simulink model "scheda_analogica_i"  (R2021a)
settings: Solver=VariableStepAuto  StartTime=0.0  StopTime=0.2  RelTol=1e-3
values from neighbouring files (symbols this model uses):
  R = 10e3    (= 10000)    [init_data.m]
  Rburden = 6.6/(1000/3000)    (= 19.8)    [init_data.m]
libraries: fl_lib x132, nesl_utility x23, ee_lib x4
settings Model: Creator=dbagn  LastModifiedBy=dbagn

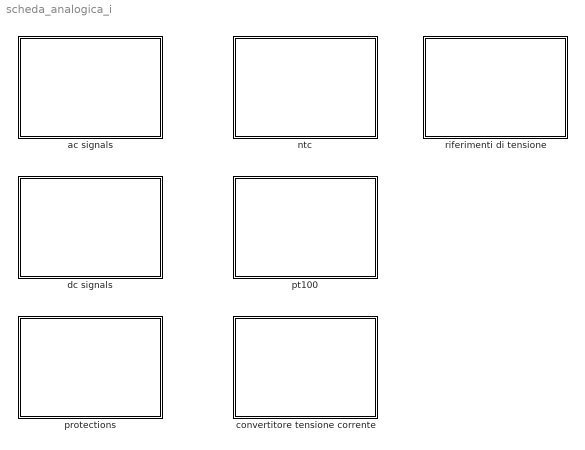
== system scheda_analogica_i ==
  ac signals : Subsystem
  convertitore tensione corrente : Subsystem
  dc signals : Subsystem
  ntc : Subsystem
  protections : Subsystem
  pt100 : Subsystem
  riferimenti di tensione : Subsystem

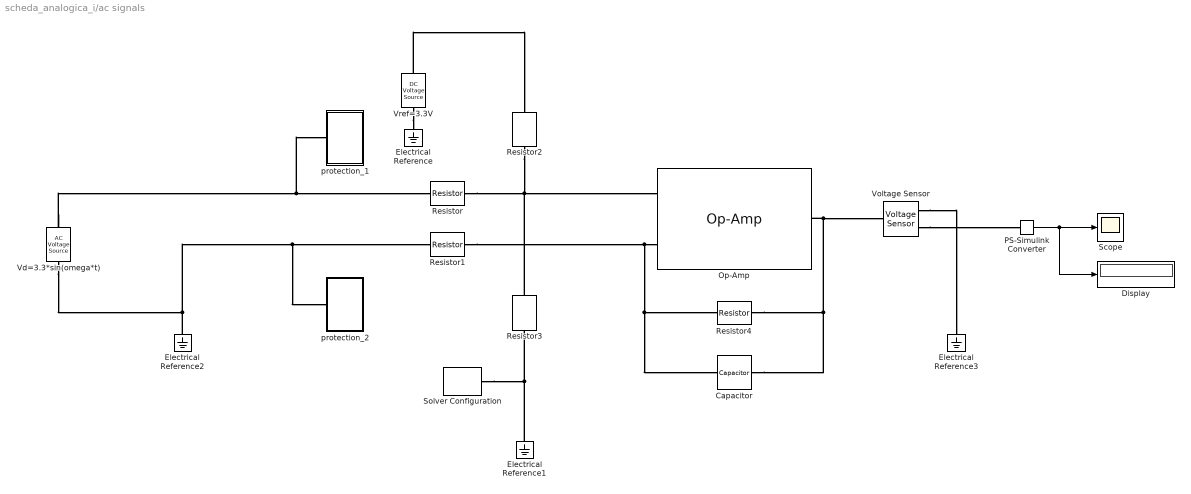
== system scheda_analogica_i/ac signals ==
  Capacitor : fl_lib/Electrical/Electrical Elements/Capacitor  c=47e-12 F  r=0 Ohm  g=0 1/Ohm  i_specify=off  i_priority=None  i=0 A  i_nominal_specify=off  i_nominal_unit=A  i_nominal_value=1  v_specify=off  v_priority=None  v=0 V  v_nominal_specify=off  v_nominal_unit=V  v_nominal_value=1  vc_specify=off  vc_priority=High  vc=0 V  vc_nominal_specify=off  vc_nominal_unit=V  vc_nominal_value=1
  Display : Display
      settings: Decimation=3
  Electrical Reference{,1..3} (4 alike) : fl_lib/Electrical/Electrical Elements/Electrical Reference
  Op-Amp : fl_lib/Electrical/Electrical Elements/Op-Amp  outI_specify=off  outI_priority=None  outI=0 A  outI_nominal_specify=off  outI_nominal_unit=A  outI_nominal_value=1
  PS-Simulink Converter : nesl_utility/PS-Simulink Converter  PhysicalDomain=network_engine_domain  SubClassName=ps_output  LeftPortType=input  RightPortType=output  PseudoPeriodic=off  Frequencies=[]  Unit=V  AffineConversion=on
      settings: SourceProductBaseCode=PW,SS
  Resistor{,1..3} (4 alike) : fl_lib/Electrical/Electrical Elements/Resistor  R=2*R Ohm  i_specify=off  i_priority=None  i=0 A  i_nominal_specify=off  i_nominal_unit=A  i_nominal_value=1  v_specify=off  v_priority=None  v=0 V  v_nominal_specify=off  v_nominal_unit=V  v_nominal_value=1
  Resistor4 : fl_lib/Electrical/Electrical Elements/Resistor  R=R Ohm  i_specify=off  i_priority=None  i=0 A  i_nominal_specify=off  i_nominal_unit=A  i_nominal_value=1  v_specify=off  v_priority=None  v=0 V  v_nominal_specify=off  v_nominal_unit=V  v_nominal_value=1
  Scope : Scope
  Solver Configuration : nesl_utility/Solver Configuration  PhysicalDomain=network_engine_domain  SubClassName=solver  LeftPortType=input  RightPortType=generic  Tones=[]  Harmonics=[]  SimulateNoise=off  Profile=off  UseLocalSampling=off  EnableSwitchedLinearOptims=on  FrequencyDomain=off  UseCCode=off  RelTol=0.001  AbsTol=1e-06  MinStep=1e-09  ToWorkspace=off  RevertToSquareIcSolve=off  NumHomotopyIterations=100  PhasorMode=off  PhasorModeNumHarmonics=1  DoDC=off  ResidualTolerance=1e-09  UseLocalSolver=off  LocalSolverChoice=NE_BACKWARD_EULER_ADVANCER  LocalSolverSampleTime=0.001  DoFixedCost=off  MaxNonlinIter=3  MaxModeIter=2  ComputeImpulses=off  ImpulseIterations=2  LinearAlgebra=auto  EquationFormulation=NE_TIME_EF  DelaysMemoryBudget=1024  AutomaticFiltering=on  FilteringTimeConstant=0.001  PartitionStorageMethod=AS_NEEDED  PartitionMemoryBudget=1024  PartitionMethod=ROBUST
      settings: SourceProductBaseCode=PW,SS
  Vd=3.3*sin(omega*t) : fl_lib/Electrical/Electrical Sources/AC Voltage Source  amp=3.3 V  shift=0 deg  frequency=50 Hz  omega=0 rad/s
  Voltage Sensor : fl_lib/Electrical/Electrical Sensors/Voltage Sensor
  Vref=3.3V : fl_lib/Electrical/Electrical Sources/DC Voltage Source  v0=3.3 V
  protection_1 : Subsystem
  protection_2 : Subsystem
  wires:
  PS-Simulink Converter/1 -> Display/1, Scope/1
  connections:
  Resistor1/RConn1 -- Capacitor/LConn1 -- Resistor4/LConn1 -- Op-Amp/LConn2
  Electrical Reference1/LConn1 -- Solver Configuration/RConn1 -- Resistor3/RConn1
  Vref=3.3V/LConn1 -- Resistor2/LConn1
  Voltage Sensor/RConn1 -- PS-Simulink Converter/LConn1
  Resistor4/RConn1 -- Op-Amp/RConn1 -- Voltage Sensor/LConn1 -- Capacitor/RConn1
  Voltage Sensor/RConn2 -- Electrical Reference3/LConn1
  Resistor3/LConn1 -- Op-Amp/LConn1 -- Resistor2/RConn1 -- Resistor/RConn1
  Vref=3.3V/RConn1 -- Electrical Reference/LConn1
  Vd=3.3*sin(omega*t)/LConn1 -- protection_1/LConn1 -- Resistor/LConn1
  Electrical Reference2/LConn1 -- Vd=3.3*sin(omega*t)/RConn1 -- protection_2/LConn1 -- Resistor1/LConn1

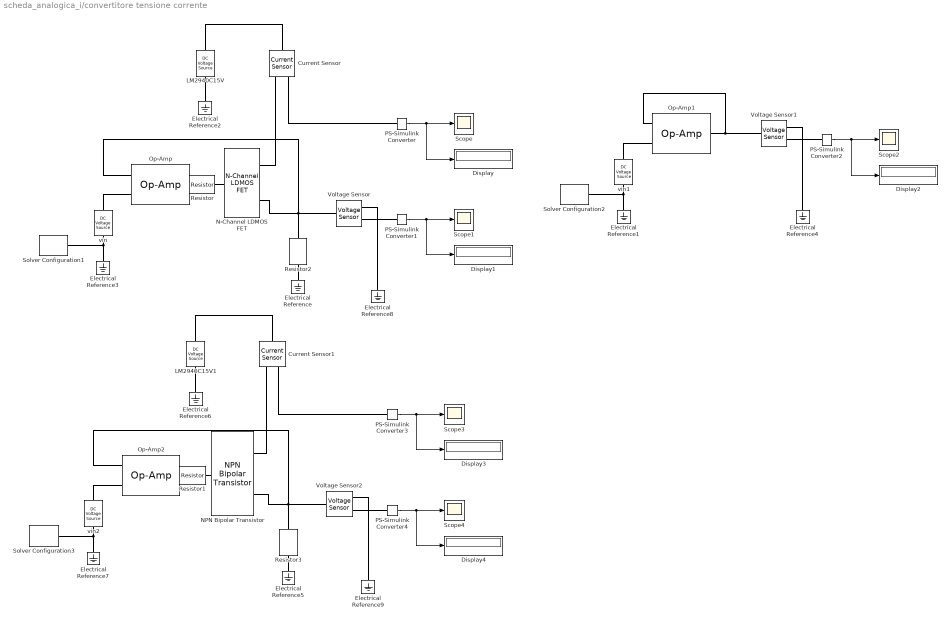
== system scheda_analogica_i/convertitore tensione corrente ==
  Current Sensor : fl_lib/Electrical/Electrical Sensors/Current Sensor
  Current Sensor1 : fl_lib/Electrical/Electrical Sensors/Current Sensor
  Display{,1..4} (5 alike) : Display
      settings: Decimation=3
  Electrical Reference{,1..9} (10 alike) : fl_lib/Electrical/Electrical Elements/Electrical Reference
  LM2940C15V : fl_lib/Electrical/Electrical Sources/DC Voltage Source  v0=15 V
  LM2940C15V1 : fl_lib/Electrical/Electrical Sources/DC Voltage Source  v0=15 V
  N-Channel LDMOS FET : ee_lib/Semiconductors & Converters/N-Channel LDMOS FET  betaref=[11.6, .01] A/V^2  Vfbref=[-1.05, -.1] V  gamma=[3.4, 2.5] V^0.50000  phib2ref=[.95, .95] V  thesatref=[0, .1] 1/V  theaccdr=0 1/V  alpha=0  Vp=5e-2 V  m=8  Tmeas=25 degC  Cox=[1600, 1000] pF  Cgso=15 pF  Cgdo=15 pF  Rsref=1e-4 Ohm  Rdref=0.07 Ohm  Rgref=8.4 Ohm  Rdriftref=0.1 Ohm  lambda=0.2  Isref=1e-13 A  Vbi=0.6 V  n=1  Cj0=1800 pF  TT=50e-9 s  Tprm=1  Tsim=25 degC  etabet=[1.3, 1.3]  Stvfb=[.0005, .0005] V/K  Stphib=-8.5e-4 V/K  etasat=[1.04, 1.04]  etar=0.95  etardr=0.95  etais=3  thermal_network_parameterization=ee.enum.thermalNetworkTopology.cauer  Rth=[0, 10] K/W  Rth_Foster=[4, 6] K/W  thermal_mass_parameterization=ee.enum.thermalNetwork.timeconstant  thermal_mass=[0, 1] J/K  thermal_mass_Foster=[1.5, 3] J/K  thermal_time_constant=[0, 10] s  thermal_time_constant_Foster=[6, 18] s  T0=[25, 25] degC
      settings: SourceProductBaseCode=PS  InternalSimscapePortConfiguration="{\"Bottom\":[],\"Left\":[{\"id\":\"G\",\"label\":\"\",\"type\":\"foundation.electrical.electrical\"}],\"Right\":[{\"id\":\"D\",\"label\":\"d\",\"type\":\"foundation.electrical.electrical\"},{\"id\":\"S\",\"label\":\"s\",\"type\":\"foundation.electrical.electrical\"}],\"Top\":[]}"
  NPN Bipolar Transistor : ee_lib/Semiconductors & Converters/NPN Bipolar Transistor  parameterization=1  prmDatasheet=1  prmEquCoeff=1  BF=100  IS=1e-14 A  VAF=200 V  hfe=100  hoe=50e-6 1/Ohm  Ic_h=1 mA  Vce_h=5 V  V1=0.55 V  I1=0.5 mA  BR=1  Tmeas=25 degC  RC=0.01 Ohm  RE=1e-4 Ohm  RB=1 Ohm  C_BC=5 pF  C_BE=5 pF  TF=0 us  TR=0 us  hfe_T2=125  XTB=0  V1_T2=0.45 V  I1_T2=0.5 mA  Tmeas2=125 degC  EG=1.11 eV  XTI=3  ec=1  TdeviceDatasheet=25 degC  TdeviceEquCoeff=25 degC  thermal_network_parameterization=ee.enum.thermalNetworkTopology.cauer  Rth=[0, 10] K/W  Rth_Foster=[4, 6] K/W  thermal_mass_parameterization=ee.enum.thermalNetwork.timeconstant  thermal_mass=[0, 1] J/K  thermal_mass_Foster=[1.5, 3] J/K  thermal_time_constant=[0, 10] s  thermal_time_constant_Foster=[6, 18] s  thermal_mass_initial_temperatures=[25, 25] degC
  Op-Amp : fl_lib/Electrical/Electrical Elements/Op-Amp  outI_specify=off  outI_priority=None  outI=0 A  outI_nominal_specify=off  outI_nominal_unit=A  outI_nominal_value=1
  Op-Amp1 : fl_lib/Electrical/Electrical Elements/Op-Amp  outI_specify=off  outI_priority=None  outI=0 A  outI_nominal_specify=off  outI_nominal_unit=A  outI_nominal_value=1
  Op-Amp2 : fl_lib/Electrical/Electrical Elements/Op-Amp  outI_specify=off  outI_priority=None  outI=0 A  outI_nominal_specify=off  outI_nominal_unit=A  outI_nominal_value=1
  PS-Simulink Converter : nesl_utility/PS-Simulink Converter  PhysicalDomain=network_engine_domain  SubClassName=ps_output  LeftPortType=input  RightPortType=output  PseudoPeriodic=off  Frequencies=[]  Unit=A  AffineConversion=on
      settings: SourceProductBaseCode=PW,SS
  PS-Simulink Converter1 : nesl_utility/PS-Simulink Converter  PhysicalDomain=network_engine_domain  SubClassName=ps_output  LeftPortType=input  RightPortType=output  PseudoPeriodic=off  Frequencies=[]  Unit=V  AffineConversion=on
      settings: SourceProductBaseCode=PW,SS
  PS-Simulink Converter2 : nesl_utility/PS-Simulink Converter  PhysicalDomain=network_engine_domain  SubClassName=ps_output  LeftPortType=input  RightPortType=output  PseudoPeriodic=off  Frequencies=[]  Unit=V  AffineConversion=on
      settings: SourceProductBaseCode=PW,SS
  PS-Simulink Converter3 : nesl_utility/PS-Simulink Converter  PhysicalDomain=network_engine_domain  SubClassName=ps_output  LeftPortType=input  RightPortType=output  PseudoPeriodic=off  Frequencies=[]  Unit=A  AffineConversion=on
      settings: SourceProductBaseCode=PW,SS
  PS-Simulink Converter4 : nesl_utility/PS-Simulink Converter  PhysicalDomain=network_engine_domain  SubClassName=ps_output  LeftPortType=input  RightPortType=output  PseudoPeriodic=off  Frequencies=[]  Unit=V  AffineConversion=on
      settings: SourceProductBaseCode=PW,SS
  Resistor{,1..3} (4 alike) : fl_lib/Electrical/Electrical Elements/Resistor  R=100 Ohm  i_specify=off  i_priority=None  i=0 A  i_nominal_specify=off  i_nominal_unit=A  i_nominal_value=1  v_specify=off  v_priority=None  v=0 V  v_nominal_specify=off  v_nominal_unit=V  v_nominal_value=1
  Scope{,1..4} (5 alike) : Scope
  Solver Configuration1 : nesl_utility/Solver Configuration  PhysicalDomain=network_engine_domain  SubClassName=solver  LeftPortType=input  RightPortType=generic  Tones=[]  Harmonics=[]  SimulateNoise=off  Profile=off  UseLocalSampling=off  EnableSwitchedLinearOptims=on  FrequencyDomain=off  UseCCode=off  RelTol=0.001  AbsTol=1e-06  MinStep=1e-09  ToWorkspace=off  RevertToSquareIcSolve=off  NumHomotopyIterations=100  PhasorMode=off  PhasorModeNumHarmonics=1  DoDC=off  ResidualTolerance=1e-09  UseLocalSolver=off  LocalSolverChoice=NE_BACKWARD_EULER_ADVANCER  LocalSolverSampleTime=0.001  DoFixedCost=off  MaxNonlinIter=3  MaxModeIter=2  ComputeImpulses=off  ImpulseIterations=2  LinearAlgebra=auto  EquationFormulation=NE_TIME_EF  DelaysMemoryBudget=1024  AutomaticFiltering=on  FilteringTimeConstant=0.001  PartitionStorageMethod=AS_NEEDED  PartitionMemoryBudget=1024  PartitionMethod=ROBUST
      settings: SourceProductBaseCode=PW,SS
  Solver Configuration2 : nesl_utility/Solver Configuration  PhysicalDomain=network_engine_domain  SubClassName=solver  LeftPortType=input  RightPortType=generic  Tones=[]  Harmonics=[]  SimulateNoise=off  Profile=off  UseLocalSampling=off  EnableSwitchedLinearOptims=on  FrequencyDomain=off  UseCCode=off  RelTol=0.001  AbsTol=1e-06  MinStep=1e-09  ToWorkspace=off  RevertToSquareIcSolve=off  NumHomotopyIterations=100  PhasorMode=off  PhasorModeNumHarmonics=1  DoDC=off  ResidualTolerance=1e-09  UseLocalSolver=off  LocalSolverChoice=NE_BACKWARD_EULER_ADVANCER  LocalSolverSampleTime=0.001  DoFixedCost=off  MaxNonlinIter=3  MaxModeIter=2  ComputeImpulses=off  ImpulseIterations=2  LinearAlgebra=auto  EquationFormulation=NE_TIME_EF  DelaysMemoryBudget=1024  AutomaticFiltering=on  FilteringTimeConstant=0.001  PartitionStorageMethod=AS_NEEDED  PartitionMemoryBudget=1024  PartitionMethod=ROBUST
      settings: SourceProductBaseCode=PW,SS
  Solver Configuration3 : nesl_utility/Solver Configuration  PhysicalDomain=network_engine_domain  SubClassName=solver  LeftPortType=input  RightPortType=generic  Tones=[]  Harmonics=[]  SimulateNoise=off  Profile=off  UseLocalSampling=off  EnableSwitchedLinearOptims=on  FrequencyDomain=off  UseCCode=off  RelTol=0.001  AbsTol=1e-06  MinStep=1e-09  ToWorkspace=off  RevertToSquareIcSolve=off  NumHomotopyIterations=100  PhasorMode=off  PhasorModeNumHarmonics=1  DoDC=off  ResidualTolerance=1e-09  UseLocalSolver=off  LocalSolverChoice=NE_BACKWARD_EULER_ADVANCER  LocalSolverSampleTime=0.001  DoFixedCost=off  MaxNonlinIter=3  MaxModeIter=2  ComputeImpulses=off  ImpulseIterations=2  LinearAlgebra=auto  EquationFormulation=NE_TIME_EF  DelaysMemoryBudget=1024  AutomaticFiltering=on  FilteringTimeConstant=0.001  PartitionStorageMethod=AS_NEEDED  PartitionMemoryBudget=1024  PartitionMethod=ROBUST
      settings: SourceProductBaseCode=PW,SS
  Voltage Sensor : fl_lib/Electrical/Electrical Sensors/Voltage Sensor
  Voltage Sensor1 : fl_lib/Electrical/Electrical Sensors/Voltage Sensor
  Voltage Sensor2 : fl_lib/Electrical/Electrical Sensors/Voltage Sensor
  vin : fl_lib/Electrical/Electrical Sources/DC Voltage Source  v0=1 V
  vin1 : fl_lib/Electrical/Electrical Sources/DC Voltage Source  v0=2.25 V
  vin2 : fl_lib/Electrical/Electrical Sources/DC Voltage Source  v0=1 V
  wires:
  PS-Simulink Converter1/1 -> Display1/1, Scope1/1
  PS-Simulink Converter/1 -> Display/1, Scope/1
  PS-Simulink Converter2/1 -> Scope2/1, Display2/1
  PS-Simulink Converter3/1 -> Scope3/1, Display3/1
  PS-Simulink Converter4/1 -> Scope4/1, Display4/1
  connections:
  Current Sensor/RConn2 -- N-Channel LDMOS FET/RConn1
  Voltage Sensor/RConn1 -- PS-Simulink Converter1/LConn1
  Voltage Sensor/RConn2 -- Electrical Reference8/LConn1
  Electrical Reference3/LConn1 -- Solver Configuration1/RConn1 -- vin/RConn1
  PS-Simulink Converter/LConn1 -- Current Sensor/RConn1
  Electrical Reference2/LConn1 -- LM2940C15V/RConn1
  Current Sensor/LConn1 -- LM2940C15V/LConn1
  vin/LConn1 -- Op-Amp/LConn1
  Voltage Sensor/LConn1 -- Resistor2/LConn1 -- N-Channel LDMOS FET/RConn2 -- Op-Amp/LConn2
  Op-Amp/RConn1 -- Resistor/LConn1
  N-Channel LDMOS FET/LConn1 -- Resistor/RConn1
  Electrical Reference/LConn1 -- Resistor2/RConn1
  Solver Configuration2/RConn1 -- Electrical Reference1/LConn1 -- vin1/RConn1
  vin1/LConn1 -- Op-Amp1/LConn1
  Op-Amp1/LConn2 -- Voltage Sensor1/LConn1 -- Op-Amp1/RConn1
  Voltage Sensor1/RConn2 -- Electrical Reference4/LConn1
  Voltage Sensor1/RConn1 -- PS-Simulink Converter2/LConn1
  Solver Configuration3/RConn1 -- Electrical Reference7/LConn1 -- vin2/RConn1
  Resistor3/LConn1 -- NPN Bipolar Transistor/RConn2 -- Op-Amp2/LConn2 -- Voltage Sensor2/LConn1
  NPN Bipolar Transistor/LConn1 -- Resistor1/RConn1
  Op-Amp2/RConn1 -- Resistor1/LConn1
  Electrical Reference6/LConn1 -- LM2940C15V1/RConn1
  PS-Simulink Converter3/LConn1 -- Current Sensor1/RConn1
  Current Sensor1/LConn1 -- LM2940C15V1/LConn1
  Electrical Reference5/LConn1 -- Resistor3/RConn1
  vin2/LConn1 -- Op-Amp2/LConn1
  Voltage Sensor2/RConn2 -- Electrical Reference9/LConn1
  Voltage Sensor2/RConn1 -- PS-Simulink Converter4/LConn1
  Current Sensor1/RConn2 -- NPN Bipolar Transistor/RConn1

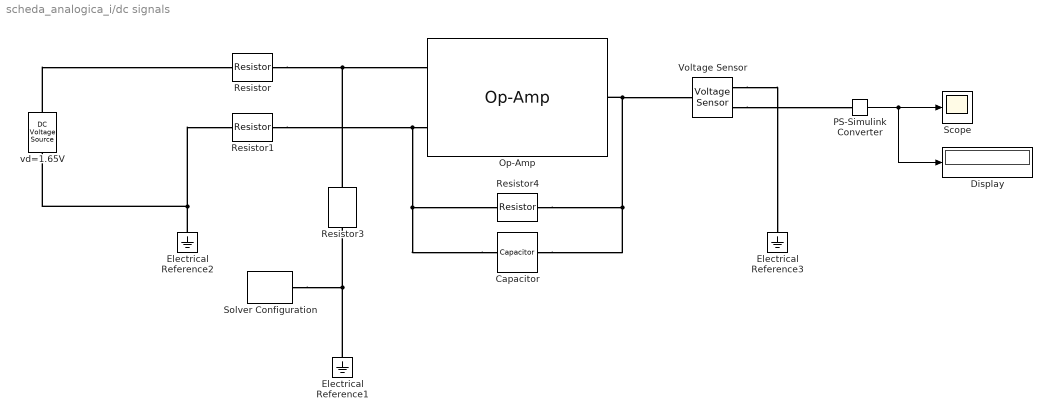
== system scheda_analogica_i/dc signals ==
  Capacitor : fl_lib/Electrical/Electrical Elements/Capacitor  c=47e-12 F  r=0 Ohm  g=0 1/Ohm  i_specify=off  i_priority=None  i=0 A  i_nominal_specify=off  i_nominal_unit=A  i_nominal_value=1  v_specify=off  v_priority=None  v=0 V  v_nominal_specify=off  v_nominal_unit=V  v_nominal_value=1  vc_specify=off  vc_priority=High  vc=0 V  vc_nominal_specify=off  vc_nominal_unit=V  vc_nominal_value=1
  Display : Display
      settings: Decimation=3
  Electrical Reference1 : fl_lib/Electrical/Electrical Elements/Electrical Reference
  Electrical Reference2 : fl_lib/Electrical/Electrical Elements/Electrical Reference
  Electrical Reference3 : fl_lib/Electrical/Electrical Elements/Electrical Reference
  Op-Amp : fl_lib/Electrical/Electrical Elements/Op-Amp  outI_specify=off  outI_priority=None  outI=0 A  outI_nominal_specify=off  outI_nominal_unit=A  outI_nominal_value=1
  PS-Simulink Converter : nesl_utility/PS-Simulink Converter  PhysicalDomain=network_engine_domain  SubClassName=ps_output  LeftPortType=input  RightPortType=output  PseudoPeriodic=off  Frequencies=[]  Unit=V  AffineConversion=on
      settings: SourceProductBaseCode=PW,SS
  Resistor : fl_lib/Electrical/Electrical Elements/Resistor  R=2*R Ohm  i_specify=off  i_priority=None  i=0 A  i_nominal_specify=off  i_nominal_unit=A  i_nominal_value=1  v_specify=off  v_priority=None  v=0 V  v_nominal_specify=off  v_nominal_unit=V  v_nominal_value=1
  Resistor1 : fl_lib/Electrical/Electrical Elements/Resistor  R=2*R Ohm  i_specify=off  i_priority=None  i=0 A  i_nominal_specify=off  i_nominal_unit=A  i_nominal_value=1  v_specify=off  v_priority=None  v=0 V  v_nominal_specify=off  v_nominal_unit=V  v_nominal_value=1
  Resistor3 : fl_lib/Electrical/Electrical Elements/Resistor  R=R Ohm  i_specify=off  i_priority=None  i=0 A  i_nominal_specify=off  i_nominal_unit=A  i_nominal_value=1  v_specify=off  v_priority=None  v=0 V  v_nominal_specify=off  v_nominal_unit=V  v_nominal_value=1
  Resistor4 : fl_lib/Electrical/Electrical Elements/Resistor  R=R Ohm  i_specify=off  i_priority=None  i=0 A  i_nominal_specify=off  i_nominal_unit=A  i_nominal_value=1  v_specify=off  v_priority=None  v=0 V  v_nominal_specify=off  v_nominal_unit=V  v_nominal_value=1
  Scope : Scope
  Solver Configuration : nesl_utility/Solver Configuration  PhysicalDomain=network_engine_domain  SubClassName=solver  LeftPortType=input  RightPortType=generic  Tones=[]  Harmonics=[]  SimulateNoise=off  Profile=off  UseLocalSampling=off  EnableSwitchedLinearOptims=on  FrequencyDomain=off  UseCCode=off  RelTol=0.001  AbsTol=1e-06  MinStep=1e-09  ToWorkspace=off  RevertToSquareIcSolve=off  NumHomotopyIterations=100  PhasorMode=off  PhasorModeNumHarmonics=1  DoDC=off  ResidualTolerance=1e-09  UseLocalSolver=off  LocalSolverChoice=NE_BACKWARD_EULER_ADVANCER  LocalSolverSampleTime=0.001  DoFixedCost=off  MaxNonlinIter=3  MaxModeIter=2  ComputeImpulses=off  ImpulseIterations=2  LinearAlgebra=auto  EquationFormulation=NE_TIME_EF  DelaysMemoryBudget=1024  AutomaticFiltering=on  FilteringTimeConstant=0.001  PartitionStorageMethod=AS_NEEDED  PartitionMemoryBudget=1024  PartitionMethod=ROBUST
      settings: SourceProductBaseCode=PW,SS
  Voltage Sensor : fl_lib/Electrical/Electrical Sensors/Voltage Sensor
  vd=1.65V : fl_lib/Electrical/Electrical Sources/DC Voltage Source  v0=1.65 V
  wires:
  PS-Simulink Converter/1 -> Scope/1, Display/1
  connections:
  Resistor3/LConn1 -- Resistor/RConn1 -- Op-Amp/LConn1
  Voltage Sensor/RConn2 -- Electrical Reference3/LConn1
  vd=1.65V/LConn1 -- Resistor/LConn1
  Capacitor/RConn1 -- Resistor4/RConn1 -- Voltage Sensor/LConn1 -- Op-Amp/RConn1
  Voltage Sensor/RConn1 -- PS-Simulink Converter/LConn1
  Solver Configuration/RConn1 -- Electrical Reference1/LConn1 -- Resistor3/RConn1
  Capacitor/LConn1 -- Resistor4/LConn1 -- Resistor1/RConn1 -- Op-Amp/LConn2
  vd=1.65V/RConn1 -- Electrical Reference2/LConn1 -- Resistor1/LConn1

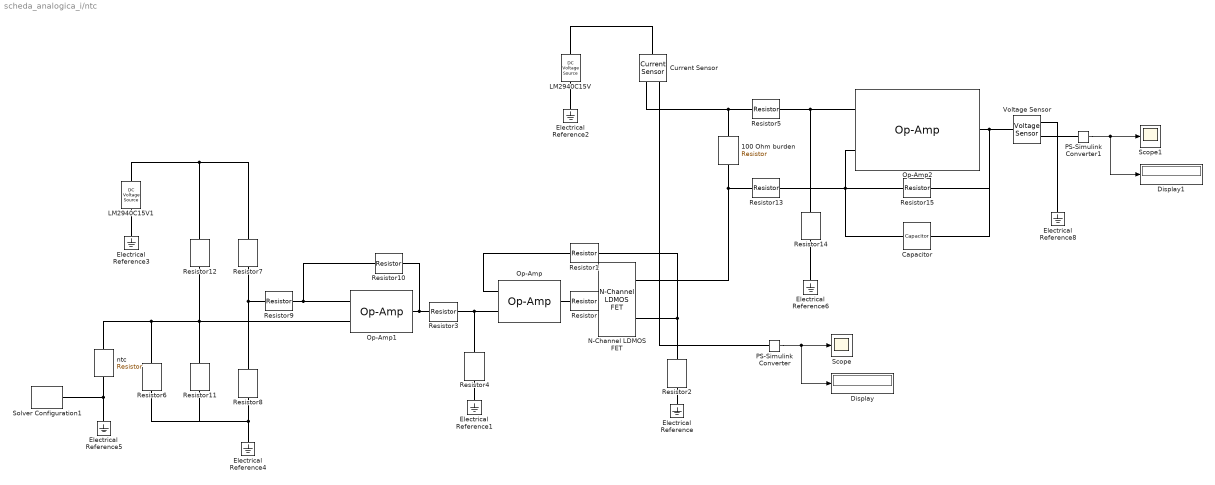
== system scheda_analogica_i/ntc ==
  100 Ohm burden : fl_lib/Electrical/Electrical Elements/Resistor  R=100 Ohm  i_specify=off  i_priority=None  i=0 A  i_nominal_specify=off  i_nominal_unit=A  i_nominal_value=1  v_specify=off  v_priority=None  v=0 V  v_nominal_specify=off  v_nominal_unit=V  v_nominal_value=1
  Capacitor : fl_lib/Electrical/Electrical Elements/Capacitor  c=47e-12 F  r=0 Ohm  g=0 1/Ohm  i_specify=off  i_priority=None  i=0 A  i_nominal_specify=off  i_nominal_unit=A  i_nominal_value=1  v_specify=off  v_priority=None  v=0 V  v_nominal_specify=off  v_nominal_unit=V  v_nominal_value=1  vc_specify=off  vc_priority=High  vc=0 V  vc_nominal_specify=off  vc_nominal_unit=V  vc_nominal_value=1
  Current Sensor : fl_lib/Electrical/Electrical Sensors/Current Sensor
  Display : Display
      settings: Decimation=3
  Display1 : Display
      settings: Decimation=3
  Electrical Reference{,1..6,8} (8 alike) : fl_lib/Electrical/Electrical Elements/Electrical Reference
  LM2940C15V : fl_lib/Electrical/Electrical Sources/DC Voltage Source  v0=15 V
  LM2940C15V1 : fl_lib/Electrical/Electrical Sources/DC Voltage Source  v0=15 V
  N-Channel LDMOS FET : ee_lib/Semiconductors & Converters/N-Channel LDMOS FET  betaref=[11.6, .01] A/V^2  Vfbref=[-1.05, -.1] V  gamma=[3.4, 2.5] V^0.50000  phib2ref=[.95, .95] V  thesatref=[0, .1] 1/V  theaccdr=0 1/V  alpha=0  Vp=5e-2 V  m=8  Tmeas=25 degC  Cox=[1600, 1000] pF  Cgso=15 pF  Cgdo=15 pF  Rsref=1e-4 Ohm  Rdref=0.07 Ohm  Rgref=8.4 Ohm  Rdriftref=0.1 Ohm  lambda=0.2  Isref=1e-13 A  Vbi=0.6 V  n=1  Cj0=1800 pF  TT=50e-9 s  Tprm=1  Tsim=25 degC  etabet=[1.3, 1.3]  Stvfb=[.0005, .0005] V/K  Stphib=-8.5e-4 V/K  etasat=[1.04, 1.04]  etar=0.95  etardr=0.95  etais=3  thermal_network_parameterization=ee.enum.thermalNetworkTopology.cauer  Rth=[0, 10] K/W  Rth_Foster=[4, 6] K/W  thermal_mass_parameterization=ee.enum.thermalNetwork.timeconstant  thermal_mass=[0, 1] J/K  thermal_mass_Foster=[1.5, 3] J/K  thermal_time_constant=[0, 10] s  thermal_time_constant_Foster=[6, 18] s  T0=[25, 25] degC
      settings: SourceProductBaseCode=PS  InternalSimscapePortConfiguration="{\"Bottom\":[],\"Left\":[{\"id\":\"G\",\"label\":\"\",\"type\":\"foundation.electrical.electrical\"}],\"Right\":[{\"id\":\"D\",\"label\":\"d\",\"type\":\"foundation.electrical.electrical\"},{\"id\":\"S\",\"label\":\"s\",\"type\":\"foundation.electrical.electrical\"}],\"Top\":[]}"
  Op-Amp : fl_lib/Electrical/Electrical Elements/Op-Amp  outI_specify=off  outI_priority=None  outI=0 A  outI_nominal_specify=off  outI_nominal_unit=A  outI_nominal_value=1
  Op-Amp1 : fl_lib/Electrical/Electrical Elements/Op-Amp  outI_specify=off  outI_priority=None  outI=0 A  outI_nominal_specify=off  outI_nominal_unit=A  outI_nominal_value=1
  Op-Amp2 : fl_lib/Electrical/Electrical Elements/Op-Amp  outI_specify=off  outI_priority=None  outI=0 A  outI_nominal_specify=off  outI_nominal_unit=A  outI_nominal_value=1
  PS-Simulink Converter : nesl_utility/PS-Simulink Converter  PhysicalDomain=network_engine_domain  SubClassName=ps_output  LeftPortType=input  RightPortType=output  PseudoPeriodic=off  Frequencies=[]  Unit=A  AffineConversion=on
      settings: SourceProductBaseCode=PW,SS
  PS-Simulink Converter1 : nesl_utility/PS-Simulink Converter  PhysicalDomain=network_engine_domain  SubClassName=ps_output  LeftPortType=input  RightPortType=output  PseudoPeriodic=off  Frequencies=[]  Unit=V  AffineConversion=on
      settings: SourceProductBaseCode=PW,SS
  Resistor : fl_lib/Electrical/Electrical Elements/Resistor  R=100 Ohm  i_specify=off  i_priority=None  i=0 A  i_nominal_specify=off  i_nominal_unit=A  i_nominal_value=1  v_specify=off  v_priority=None  v=0 V  v_nominal_specify=off  v_nominal_unit=V  v_nominal_value=1
  Resistor1 : fl_lib/Electrical/Electrical Elements/Resistor  R=1e3 Ohm  i_specify=off  i_priority=None  i=0 A  i_nominal_specify=off  i_nominal_unit=A  i_nominal_value=1  v_specify=off  v_priority=None  v=0 V  v_nominal_specify=off  v_nominal_unit=V  v_nominal_value=1
  Resistor10 : fl_lib/Electrical/Electrical Elements/Resistor  R=5.6e3 Ohm  i_specify=off  i_priority=None  i=0 A  i_nominal_specify=off  i_nominal_unit=A  i_nominal_value=1  v_specify=off  v_priority=None  v=0 V  v_nominal_specify=off  v_nominal_unit=V  v_nominal_value=1
  Resistor11 : fl_lib/Electrical/Electrical Elements/Resistor  R=120e3 Ohm  i_specify=off  i_priority=None  i=0 A  i_nominal_specify=off  i_nominal_unit=A  i_nominal_value=1  v_specify=off  v_priority=None  v=0 V  v_nominal_specify=off  v_nominal_unit=V  v_nominal_value=1
  Resistor12 : fl_lib/Electrical/Electrical Elements/Resistor  R=8.66e3 Ohm  i_specify=off  i_priority=None  i=0 A  i_nominal_specify=off  i_nominal_unit=A  i_nominal_value=1  v_specify=off  v_priority=None  v=0 V  v_nominal_specify=off  v_nominal_unit=V  v_nominal_value=1
  Resistor13 : fl_lib/Electrical/Electrical Elements/Resistor  R=15.4e3 Ohm  i_specify=off  i_priority=None  i=0 A  i_nominal_specify=off  i_nominal_unit=A  i_nominal_value=1  v_specify=off  v_priority=None  v=0 V  v_nominal_specify=off  v_nominal_unit=V  v_nominal_value=1
  Resistor14 : fl_lib/Electrical/Electrical Elements/Resistor  R=10e3 Ohm  i_specify=off  i_priority=None  i=0 A  i_nominal_specify=off  i_nominal_unit=A  i_nominal_value=1  v_specify=off  v_priority=None  v=0 V  v_nominal_specify=off  v_nominal_unit=V  v_nominal_value=1
  Resistor15 : fl_lib/Electrical/Electrical Elements/Resistor  R=10e3 Ohm  i_specify=off  i_priority=None  i=0 A  i_nominal_specify=off  i_nominal_unit=A  i_nominal_value=1  v_specify=off  v_priority=None  v=0 V  v_nominal_specify=off  v_nominal_unit=V  v_nominal_value=1
  Resistor2 : fl_lib/Electrical/Electrical Elements/Resistor  R=100 Ohm  i_specify=off  i_priority=None  i=0 A  i_nominal_specify=off  i_nominal_unit=A  i_nominal_value=1  v_specify=off  v_priority=None  v=0 V  v_nominal_specify=off  v_nominal_unit=V  v_nominal_value=1
  Resistor3 : fl_lib/Electrical/Electrical Elements/Resistor  R=10e3 Ohm  i_specify=off  i_priority=None  i=0 A  i_nominal_specify=off  i_nominal_unit=A  i_nominal_value=1  v_specify=off  v_priority=None  v=0 V  v_nominal_specify=off  v_nominal_unit=V  v_nominal_value=1
  Resistor4 : fl_lib/Electrical/Electrical Elements/Resistor  R=4.7e3 Ohm  i_specify=off  i_priority=None  i=0 A  i_nominal_specify=off  i_nominal_unit=A  i_nominal_value=1  v_specify=off  v_priority=None  v=0 V  v_nominal_specify=off  v_nominal_unit=V  v_nominal_value=1
  Resistor5 : fl_lib/Electrical/Electrical Elements/Resistor  R=15.4e3 Ohm  i_specify=off  i_priority=None  i=0 A  i_nominal_specify=off  i_nominal_unit=A  i_nominal_value=1  v_specify=off  v_priority=None  v=0 V  v_nominal_specify=off  v_nominal_unit=V  v_nominal_value=1
  Resistor6 : fl_lib/Electrical/Electrical Elements/Resistor  R=1.5e3 Ohm  i_specify=off  i_priority=None  i=0 A  i_nominal_specify=off  i_nominal_unit=A  i_nominal_value=1  v_specify=off  v_priority=None  v=0 V  v_nominal_specify=off  v_nominal_unit=V  v_nominal_value=1
  Resistor7 : fl_lib/Electrical/Electrical Elements/Resistor  R=33e3 Ohm  i_specify=off  i_priority=None  i=0 A  i_nominal_specify=off  i_nominal_unit=A  i_nominal_value=1  v_specify=off  v_priority=None  v=0 V  v_nominal_specify=off  v_nominal_unit=V  v_nominal_value=1
  Resistor8 : fl_lib/Electrical/Electrical Elements/Resistor  R=100 Ohm  i_specify=off  i_priority=None  i=0 A  i_nominal_specify=off  i_nominal_unit=A  i_nominal_value=1  v_specify=off  v_priority=None  v=0 V  v_nominal_specify=off  v_nominal_unit=V  v_nominal_value=1
  Resistor9 : fl_lib/Electrical/Electrical Elements/Resistor  R=1e3 Ohm  i_specify=off  i_priority=None  i=0 A  i_nominal_specify=off  i_nominal_unit=A  i_nominal_value=1  v_specify=off  v_priority=None  v=0 V  v_nominal_specify=off  v_nominal_unit=V  v_nominal_value=1
  Scope : Scope
  Scope1 : Scope
  Solver Configuration1 : nesl_utility/Solver Configuration  PhysicalDomain=network_engine_domain  SubClassName=solver  LeftPortType=input  RightPortType=generic  Tones=[]  Harmonics=[]  SimulateNoise=off  Profile=off  UseLocalSampling=off  EnableSwitchedLinearOptims=on  FrequencyDomain=off  UseCCode=off  RelTol=0.001  AbsTol=1e-06  MinStep=1e-09  ToWorkspace=off  RevertToSquareIcSolve=off  NumHomotopyIterations=100  PhasorMode=off  PhasorModeNumHarmonics=1  DoDC=off  ResidualTolerance=1e-09  UseLocalSolver=off  LocalSolverChoice=NE_BACKWARD_EULER_ADVANCER  LocalSolverSampleTime=0.001  DoFixedCost=off  MaxNonlinIter=3  MaxModeIter=2  ComputeImpulses=off  ImpulseIterations=2  LinearAlgebra=auto  EquationFormulation=NE_TIME_EF  DelaysMemoryBudget=1024  AutomaticFiltering=on  FilteringTimeConstant=0.001  PartitionStorageMethod=AS_NEEDED  PartitionMemoryBudget=1024  PartitionMethod=ROBUST
      settings: SourceProductBaseCode=PW,SS
  Voltage Sensor : fl_lib/Electrical/Electrical Sensors/Voltage Sensor
  ntc : fl_lib/Electrical/Electrical Elements/Resistor  R=120 Ohm  i_specify=off  i_priority=None  i=0 A  i_nominal_specify=off  i_nominal_unit=A  i_nominal_value=1  v_specify=off  v_priority=None  v=0 V  v_nominal_specify=off  v_nominal_unit=V  v_nominal_value=1
  wires:
  PS-Simulink Converter/1 -> Scope/1, Display/1
  PS-Simulink Converter1/1 -> Scope1/1, Display1/1
  connections:
  Current Sensor/RConn2 -- Resistor5/LConn1 -- 100 Ohm burden/LConn1
  Electrical Reference/LConn1 -- Resistor2/RConn1
  N-Channel LDMOS FET/LConn1 -- Resistor/RConn1
  Op-Amp/RConn1 -- Resistor/LConn1
  Resistor1/LConn1 -- Op-Amp/LConn2
  Resistor1/RConn1 -- N-Channel LDMOS FET/RConn2 -- Resistor2/LConn1
  Resistor3/RConn1 -- Resistor4/LConn1 -- Op-Amp/LConn1
  Electrical Reference1/LConn1 -- Resistor4/RConn1
  Current Sensor/LConn1 -- LM2940C15V/LConn1
  Electrical Reference2/LConn1 -- LM2940C15V/RConn1
  PS-Simulink Converter/LConn1 -- Current Sensor/RConn1
  Electrical Reference3/LConn1 -- LM2940C15V1/RConn1
  Resistor7/LConn1 -- Resistor12/LConn1 -- LM2940C15V1/LConn1
  Resistor8/LConn1 -- Resistor9/LConn1 -- Resistor7/RConn1
  Resistor9/RConn1 -- Resistor10/LConn1 -- Op-Amp1/LConn2
  Resistor10/RConn1 -- Op-Amp1/RConn1 -- Resistor3/LConn1
  Resistor11/LConn1 -- Resistor12/RConn1 -- ntc/LConn1 -- Resistor6/LConn1 -- Op-Amp1/LConn1
  Electrical Reference4/LConn1 -- Resistor6/RConn1 -- Resistor11/RConn1 -- Resistor8/RConn1
  Electrical Reference5/LConn1 -- Solver Configuration1/RConn1 -- ntc/RConn1
  Resistor5/RConn1 -- Resistor14/LConn1 -- Op-Amp2/LConn1
  Resistor13/RConn1 -- Capacitor/LConn1 -- Resistor15/LConn1 -- Op-Amp2/LConn2
  Op-Amp2/RConn1 -- Resistor15/RConn1 -- Capacitor/RConn1 -- Voltage Sensor/LConn1
  Voltage Sensor/RConn2 -- Electrical Reference8/LConn1
  Voltage Sensor/RConn1 -- PS-Simulink Converter1/LConn1
  100 Ohm burden/RConn1 -- Resistor13/LConn1 -- N-Channel LDMOS FET/RConn1
  Electrical Reference6/LConn1 -- Resistor14/RConn1

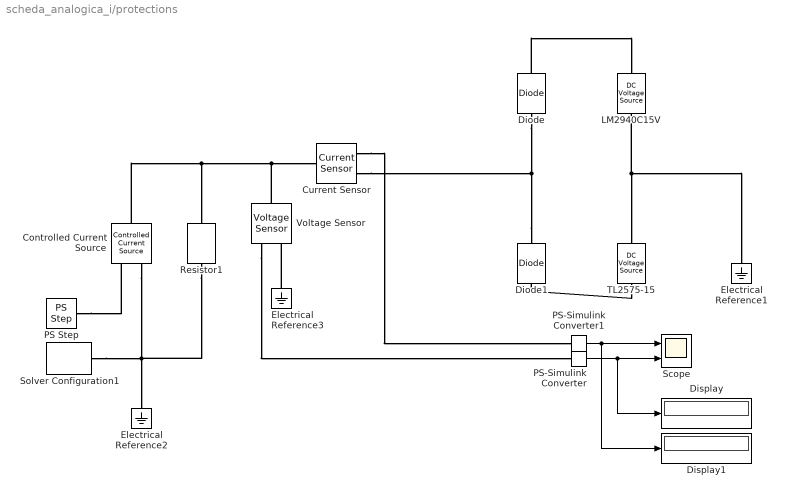
== system scheda_analogica_i/protections ==
  Controlled Current Source : fl_lib/Electrical/Electrical Sources/Controlled Current Source
  Current Sensor : fl_lib/Electrical/Electrical Sensors/Current Sensor
  Diode : fl_lib/Electrical/Electrical Elements/Diode  Vf=0.6 V  Ron=0.3 Ohm  Goff=1e-8 1/Ohm  i_specify=off  i_priority=None  i=0 A  i_nominal_specify=off  i_nominal_unit=A  i_nominal_value=1  v_specify=off  v_priority=None  v=0 V  v_nominal_specify=off  v_nominal_unit=V  v_nominal_value=1
  Diode1 : fl_lib/Electrical/Electrical Elements/Diode  Vf=0.6 V  Ron=0.3 Ohm  Goff=1e-8 1/Ohm  i_specify=off  i_priority=None  i=0 A  i_nominal_specify=off  i_nominal_unit=A  i_nominal_value=1  v_specify=off  v_priority=None  v=0 V  v_nominal_specify=off  v_nominal_unit=V  v_nominal_value=1
  Display : Display
      settings: Decimation=3
  Display1 : Display
      settings: Decimation=3
  Electrical Reference1 : fl_lib/Electrical/Electrical Elements/Electrical Reference
  Electrical Reference2 : fl_lib/Electrical/Electrical Elements/Electrical Reference
  Electrical Reference3 : fl_lib/Electrical/Electrical Elements/Electrical Reference
  LM2940C15V : fl_lib/Electrical/Electrical Sources/DC Voltage Source  v0=15 V
  PS Step : fl_lib/Physical Signals/Sources/PS Step  step_time=0.1 s  initial_value=0.3 A  final_value=2 A
      settings: SourceProductBaseCode=SS
  PS-Simulink Converter : nesl_utility/PS-Simulink Converter  PhysicalDomain=network_engine_domain  SubClassName=ps_output  LeftPortType=input  RightPortType=output  PseudoPeriodic=off  Frequencies=[]  Unit=V  AffineConversion=on
      settings: SourceProductBaseCode=PW,SS
  PS-Simulink Converter1 : nesl_utility/PS-Simulink Converter  PhysicalDomain=network_engine_domain  SubClassName=ps_output  LeftPortType=input  RightPortType=output  PseudoPeriodic=off  Frequencies=[]  Unit=A  AffineConversion=on
      settings: SourceProductBaseCode=PW,SS
  Resistor1 : fl_lib/Electrical/Electrical Elements/Resistor  R=Rburden Ohm  i_specify=off  i_priority=None  i=0 A  i_nominal_specify=off  i_nominal_unit=A  i_nominal_value=1  v_specify=off  v_priority=None  v=0 V  v_nominal_specify=off  v_nominal_unit=V  v_nominal_value=1
  Scope : Scope  NumInputPorts=2
  Solver Configuration1 : nesl_utility/Solver Configuration  PhysicalDomain=network_engine_domain  SubClassName=solver  LeftPortType=input  RightPortType=generic  Tones=[]  Harmonics=[]  SimulateNoise=off  Profile=off  UseLocalSampling=off  EnableSwitchedLinearOptims=on  FrequencyDomain=off  UseCCode=off  RelTol=0.001  AbsTol=1e-06  MinStep=1e-09  ToWorkspace=off  RevertToSquareIcSolve=off  NumHomotopyIterations=100  PhasorMode=off  PhasorModeNumHarmonics=1  DoDC=off  ResidualTolerance=1e-09  UseLocalSolver=off  LocalSolverChoice=NE_BACKWARD_EULER_ADVANCER  LocalSolverSampleTime=0.001  DoFixedCost=off  MaxNonlinIter=3  MaxModeIter=2  ComputeImpulses=off  ImpulseIterations=2  LinearAlgebra=auto  EquationFormulation=NE_TIME_EF  DelaysMemoryBudget=1024  AutomaticFiltering=on  FilteringTimeConstant=0.001  PartitionStorageMethod=AS_NEEDED  PartitionMemoryBudget=1024  PartitionMethod=ROBUST
      settings: SourceProductBaseCode=PW,SS
  TL2575-15 : fl_lib/Electrical/Electrical Sources/DC Voltage Source  v0=15 V
  Voltage Sensor : fl_lib/Electrical/Electrical Sensors/Voltage Sensor
  wires:
  PS-Simulink Converter/1 -> Scope/2, Display/1
  PS-Simulink Converter1/1 -> Display1/1, Scope/1
  connections:
  Voltage Sensor/RConn1 -- PS-Simulink Converter/LConn1
  Current Sensor/RConn1 -- PS-Simulink Converter1/LConn1
  PS Step/RConn1 -- Controlled Current Source/RConn1
  Controlled Current Source/RConn2 -- Resistor1/RConn1 -- Solver Configuration1/RConn1 -- Electrical Reference2/LConn1
  Controlled Current Source/LConn1 -- Voltage Sensor/LConn1 -- Current Sensor/LConn1 -- Resistor1/LConn1
  LM2940C15V/RConn1 -- TL2575-15/LConn1 -- Electrical Reference1/LConn1
  TL2575-15/RConn1 -- Diode1/LConn1
  Electrical Reference3/LConn1 -- Voltage Sensor/RConn2
  Diode/RConn1 -- LM2940C15V/LConn1
  Diode1/RConn1 -- Current Sensor/RConn2 -- Diode/LConn1

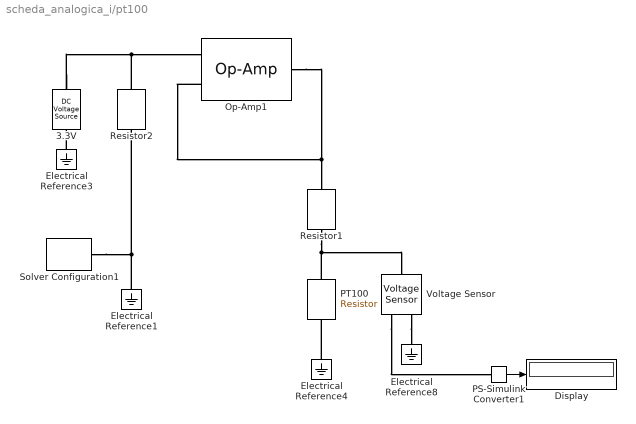
== system scheda_analogica_i/pt100 ==
  3.3V : fl_lib/Electrical/Electrical Sources/DC Voltage Source  v0=3.3 V
  Display : Display
      settings: Decimation=3
  Electrical Reference{1,3..4,8} (4 alike) : fl_lib/Electrical/Electrical Elements/Electrical Reference
  Op-Amp1 : fl_lib/Electrical/Electrical Elements/Op-Amp  outI_specify=off  outI_priority=None  outI=0 A  outI_nominal_specify=off  outI_nominal_unit=A  outI_nominal_value=1
  PS-Simulink Converter1 : nesl_utility/PS-Simulink Converter  PhysicalDomain=network_engine_domain  SubClassName=ps_output  LeftPortType=input  RightPortType=output  PseudoPeriodic=off  Frequencies=[]  Unit=V  AffineConversion=on
      settings: SourceProductBaseCode=PW,SS
  PT100 : fl_lib/Electrical/Electrical Elements/Resistor  R=160 Ohm  i_specify=off  i_priority=None  i=0 A  i_nominal_specify=off  i_nominal_unit=A  i_nominal_value=1  v_specify=off  v_priority=None  v=0 V  v_nominal_specify=off  v_nominal_unit=V  v_nominal_value=1
  Resistor1 : fl_lib/Electrical/Electrical Elements/Resistor  R=1e3 Ohm  i_specify=off  i_priority=None  i=0 A  i_nominal_specify=off  i_nominal_unit=A  i_nominal_value=1  v_specify=off  v_priority=None  v=0 V  v_nominal_specify=off  v_nominal_unit=V  v_nominal_value=1
  Resistor2 : fl_lib/Electrical/Electrical Elements/Resistor  R=1e4 Ohm  i_specify=off  i_priority=None  i=0 A  i_nominal_specify=off  i_nominal_unit=A  i_nominal_value=1  v_specify=off  v_priority=None  v=0 V  v_nominal_specify=off  v_nominal_unit=V  v_nominal_value=1
  Solver Configuration1 : nesl_utility/Solver Configuration  PhysicalDomain=network_engine_domain  SubClassName=solver  LeftPortType=input  RightPortType=generic  Tones=[]  Harmonics=[]  SimulateNoise=off  Profile=off  UseLocalSampling=off  EnableSwitchedLinearOptims=on  FrequencyDomain=off  UseCCode=off  RelTol=0.001  AbsTol=1e-06  MinStep=1e-09  ToWorkspace=off  RevertToSquareIcSolve=off  NumHomotopyIterations=100  PhasorMode=off  PhasorModeNumHarmonics=1  DoDC=off  ResidualTolerance=1e-09  UseLocalSolver=off  LocalSolverChoice=NE_BACKWARD_EULER_ADVANCER  LocalSolverSampleTime=0.001  DoFixedCost=off  MaxNonlinIter=3  MaxModeIter=2  ComputeImpulses=off  ImpulseIterations=2  LinearAlgebra=auto  EquationFormulation=NE_TIME_EF  DelaysMemoryBudget=1024  AutomaticFiltering=on  FilteringTimeConstant=0.001  PartitionStorageMethod=AS_NEEDED  PartitionMemoryBudget=1024  PartitionMethod=ROBUST
      settings: SourceProductBaseCode=PW,SS
  Voltage Sensor : fl_lib/Electrical/Electrical Sensors/Voltage Sensor
  wires:
  PS-Simulink Converter1/1 -> Display/1
  connections:
  Electrical Reference3/LConn1 -- 3.3V/RConn1
  Op-Amp1/RConn1 -- Op-Amp1/LConn2 -- Resistor1/LConn1
  Voltage Sensor/RConn2 -- Electrical Reference8/LConn1
  Voltage Sensor/RConn1 -- PS-Simulink Converter1/LConn1
  Resistor1/RConn1 -- PT100/LConn1 -- Voltage Sensor/LConn1
  Electrical Reference4/LConn1 -- PT100/RConn1
  Resistor2/LConn1 -- 3.3V/LConn1 -- Op-Amp1/LConn1
  Electrical Reference1/LConn1 -- Solver Configuration1/RConn1 -- Resistor2/RConn1

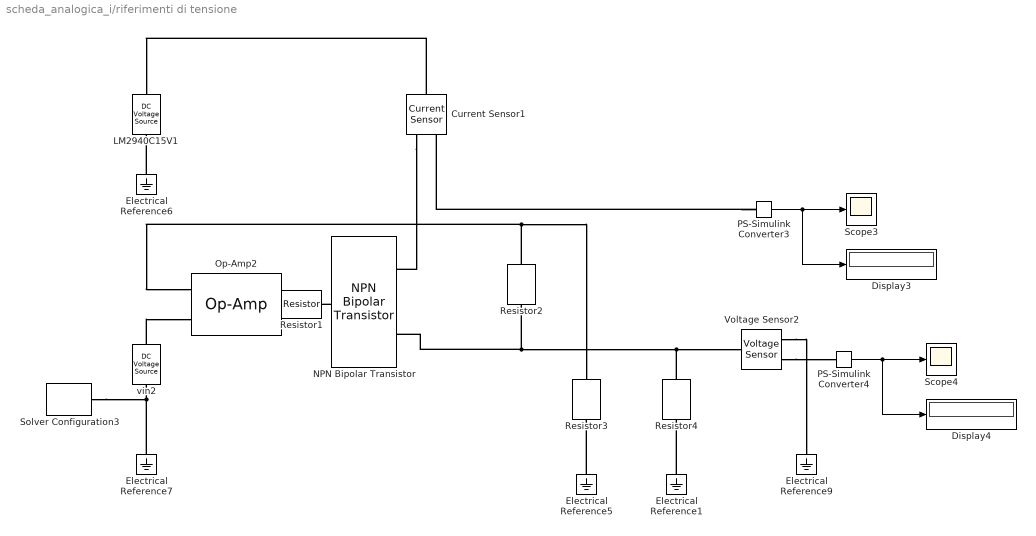
== system scheda_analogica_i/riferimenti di tensione ==
  Current Sensor1 : fl_lib/Electrical/Electrical Sensors/Current Sensor
  Display3 : Display
      settings: Decimation=3
  Display4 : Display
      settings: Decimation=3
  Electrical Reference{1,5..7,9} (5 alike) : fl_lib/Electrical/Electrical Elements/Electrical Reference
  LM2940C15V1 : fl_lib/Electrical/Electrical Sources/DC Voltage Source  v0=15 V
  NPN Bipolar Transistor : ee_lib/Semiconductors & Converters/NPN Bipolar Transistor  parameterization=1  prmDatasheet=1  prmEquCoeff=1  BF=100  IS=1e-14 A  VAF=200 V  hfe=100  hoe=50e-6 1/Ohm  Ic_h=1 mA  Vce_h=5 V  V1=0.55 V  I1=0.5 mA  BR=1  Tmeas=25 degC  RC=0.01 Ohm  RE=1e-4 Ohm  RB=1 Ohm  C_BC=5 pF  C_BE=5 pF  TF=0 us  TR=0 us  hfe_T2=125  XTB=0  V1_T2=0.45 V  I1_T2=0.5 mA  Tmeas2=125 degC  EG=1.11 eV  XTI=3  ec=1  TdeviceDatasheet=25 degC  TdeviceEquCoeff=25 degC  thermal_network_parameterization=ee.enum.thermalNetworkTopology.cauer  Rth=[0, 10] K/W  Rth_Foster=[4, 6] K/W  thermal_mass_parameterization=ee.enum.thermalNetwork.timeconstant  thermal_mass=[0, 1] J/K  thermal_mass_Foster=[1.5, 3] J/K  thermal_time_constant=[0, 10] s  thermal_time_constant_Foster=[6, 18] s  thermal_mass_initial_temperatures=[25, 25] degC
  Op-Amp2 : fl_lib/Electrical/Electrical Elements/Op-Amp  outI_specify=off  outI_priority=None  outI=0 A  outI_nominal_specify=off  outI_nominal_unit=A  outI_nominal_value=1
  PS-Simulink Converter3 : nesl_utility/PS-Simulink Converter  PhysicalDomain=network_engine_domain  SubClassName=ps_output  LeftPortType=input  RightPortType=output  PseudoPeriodic=off  Frequencies=[]  Unit=A  AffineConversion=on
      settings: SourceProductBaseCode=PW,SS
  PS-Simulink Converter4 : nesl_utility/PS-Simulink Converter  PhysicalDomain=network_engine_domain  SubClassName=ps_output  LeftPortType=input  RightPortType=output  PseudoPeriodic=off  Frequencies=[]  Unit=V  AffineConversion=on
      settings: SourceProductBaseCode=PW,SS
  Resistor1 : fl_lib/Electrical/Electrical Elements/Resistor  R=100 Ohm  i_specify=off  i_priority=None  i=0 A  i_nominal_specify=off  i_nominal_unit=A  i_nominal_value=1  v_specify=off  v_priority=None  v=0 V  v_nominal_specify=off  v_nominal_unit=V  v_nominal_value=1
  Resistor2 : fl_lib/Electrical/Electrical Elements/Resistor  R=10e3 Ohm  i_specify=off  i_priority=None  i=0 A  i_nominal_specify=off  i_nominal_unit=A  i_nominal_value=1  v_specify=off  v_priority=None  v=0 V  v_nominal_specify=off  v_nominal_unit=V  v_nominal_value=1
  Resistor3 : fl_lib/Electrical/Electrical Elements/Resistor  R=10e3 Ohm  i_specify=off  i_priority=None  i=0 A  i_nominal_specify=off  i_nominal_unit=A  i_nominal_value=1  v_specify=off  v_priority=None  v=0 V  v_nominal_specify=off  v_nominal_unit=V  v_nominal_value=1
  Resistor4 : fl_lib/Electrical/Electrical Elements/Resistor  R=5 Ohm  i_specify=off  i_priority=None  i=0 A  i_nominal_specify=off  i_nominal_unit=A  i_nominal_value=1  v_specify=off  v_priority=None  v=0 V  v_nominal_specify=off  v_nominal_unit=V  v_nominal_value=1
  Scope3 : Scope
  Scope4 : Scope
  Solver Configuration3 : nesl_utility/Solver Configuration  PhysicalDomain=network_engine_domain  SubClassName=solver  LeftPortType=input  RightPortType=generic  Tones=[]  Harmonics=[]  SimulateNoise=off  Profile=off  UseLocalSampling=off  EnableSwitchedLinearOptims=on  FrequencyDomain=off  UseCCode=off  RelTol=0.001  AbsTol=1e-06  MinStep=1e-09  ToWorkspace=off  RevertToSquareIcSolve=off  NumHomotopyIterations=100  PhasorMode=off  PhasorModeNumHarmonics=1  DoDC=off  ResidualTolerance=1e-09  UseLocalSolver=off  LocalSolverChoice=NE_BACKWARD_EULER_ADVANCER  LocalSolverSampleTime=0.001  DoFixedCost=off  MaxNonlinIter=3  MaxModeIter=2  ComputeImpulses=off  ImpulseIterations=2  LinearAlgebra=auto  EquationFormulation=NE_TIME_EF  DelaysMemoryBudget=1024  AutomaticFiltering=on  FilteringTimeConstant=0.001  PartitionStorageMethod=AS_NEEDED  PartitionMemoryBudget=1024  PartitionMethod=ROBUST
      settings: SourceProductBaseCode=PW,SS
  Voltage Sensor2 : fl_lib/Electrical/Electrical Sensors/Voltage Sensor
  vin2 : fl_lib/Electrical/Electrical Sources/DC Voltage Source  v0=2.5 V
  wires:
  PS-Simulink Converter4/1 -> Display4/1, Scope4/1
  PS-Simulink Converter3/1 -> Display3/1, Scope3/1
  connections:
  Current Sensor1/RConn2 -- NPN Bipolar Transistor/RConn1
  Voltage Sensor2/RConn1 -- PS-Simulink Converter4/LConn1
  Voltage Sensor2/RConn2 -- Electrical Reference9/LConn1
  vin2/LConn1 -- Op-Amp2/LConn1
  Electrical Reference5/LConn1 -- Resistor3/RConn1
  Current Sensor1/LConn1 -- LM2940C15V1/LConn1
  PS-Simulink Converter3/LConn1 -- Current Sensor1/RConn1
  Electrical Reference6/LConn1 -- LM2940C15V1/RConn1
  Op-Amp2/RConn1 -- Resistor1/LConn1
  NPN Bipolar Transistor/LConn1 -- Resistor1/RConn1
  NPN Bipolar Transistor/RConn2 -- Resistor4/LConn1 -- Voltage Sensor2/LConn1 -- Resistor2/RConn1
  Electrical Reference7/LConn1 -- Solver Configuration3/RConn1 -- vin2/RConn1
  Resistor2/LConn1 -- Op-Amp2/LConn2 -- Resistor3/LConn1
  Electrical Reference1/LConn1 -- Resistor4/RConn1

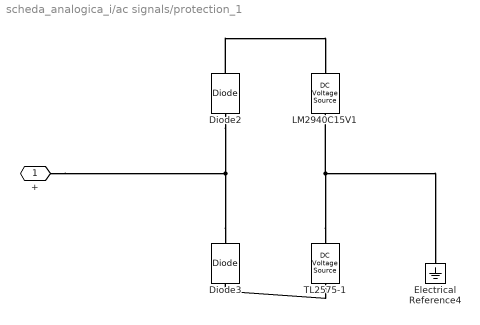
== system scheda_analogica_i/ac signals/protection_1 ==
  Diode2 : fl_lib/Electrical/Electrical Elements/Diode  Vf=0.6 V  Ron=0.3 Ohm  Goff=1e-8 1/Ohm  i_specify=off  i_priority=None  i=0 A  i_nominal_specify=off  i_nominal_unit=A  i_nominal_value=1  v_specify=off  v_priority=None  v=0 V  v_nominal_specify=off  v_nominal_unit=V  v_nominal_value=1
  Diode3 : fl_lib/Electrical/Electrical Elements/Diode  Vf=0.6 V  Ron=0.3 Ohm  Goff=1e-8 1/Ohm  i_specify=off  i_priority=None  i=0 A  i_nominal_specify=off  i_nominal_unit=A  i_nominal_value=1  v_specify=off  v_priority=None  v=0 V  v_nominal_specify=off  v_nominal_unit=V  v_nominal_value=1
  Electrical Reference4 : fl_lib/Electrical/Electrical Elements/Electrical Reference
  LM2940C15V1 : fl_lib/Electrical/Electrical Sources/DC Voltage Source  v0=15 V
  TL2575-1 : fl_lib/Electrical/Electrical Sources/DC Voltage Source  v0=15 V
  + : PMIOPort  Side=Left
  connections:
  TL2575-1/LConn1 -- Electrical Reference4/LConn1 -- LM2940C15V1/RConn1
  Diode3/RConn1 -- Diode2/LConn1 -- +/RConn1
  TL2575-1/RConn1 -- Diode3/LConn1
  Diode2/RConn1 -- LM2940C15V1/LConn1

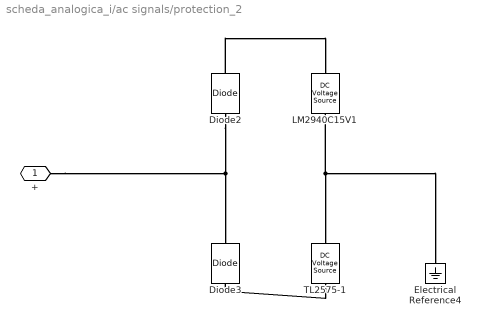
== system scheda_analogica_i/ac signals/protection_2 ==
  Diode2 : fl_lib/Electrical/Electrical Elements/Diode  Vf=0.6 V  Ron=0.3 Ohm  Goff=1e-8 1/Ohm  i_specify=off  i_priority=None  i=0 A  i_nominal_specify=off  i_nominal_unit=A  i_nominal_value=1  v_specify=off  v_priority=None  v=0 V  v_nominal_specify=off  v_nominal_unit=V  v_nominal_value=1
  Diode3 : fl_lib/Electrical/Electrical Elements/Diode  Vf=0.6 V  Ron=0.3 Ohm  Goff=1e-8 1/Ohm  i_specify=off  i_priority=None  i=0 A  i_nominal_specify=off  i_nominal_unit=A  i_nominal_value=1  v_specify=off  v_priority=None  v=0 V  v_nominal_specify=off  v_nominal_unit=V  v_nominal_value=1
  Electrical Reference4 : fl_lib/Electrical/Electrical Elements/Electrical Reference
  LM2940C15V1 : fl_lib/Electrical/Electrical Sources/DC Voltage Source  v0=15 V
  TL2575-1 : fl_lib/Electrical/Electrical Sources/DC Voltage Source  v0=15 V
  + : PMIOPort  Side=Left
  connections:
  Diode2/RConn1 -- LM2940C15V1/LConn1
  TL2575-1/RConn1 -- Diode3/LConn1
  +/RConn1 -- Diode2/LConn1 -- Diode3/RConn1
  LM2940C15V1/RConn1 -- Electrical Reference4/LConn1 -- TL2575-1/LConn1
